simulink model "fs"  (R2020a)
settings: Solver=ode4  StartTime=0.0  StopTime=inf  FixedStep=0.05  RelTol=1e-3
undefined symbols (not defined in the file): Angular, Discrete, Linear, Time
libraries: robotlib x17, simulink x1, ctrlSharedLib x1, dspstat3 x1
settings Model: Creator=ivory  LastModifiedBy=ivory
settings OptimizationCC: EnhancedBackFolding=on  PassReuseOutputArgsAs=Individual arguments  ZeroExternalMemoryAtStartup=off  ZeroInternalMemoryAtStartup=off  MaxStackSize=64  OptimizeBlockOrder=speed  DifferentSizesBufferReuse=on  OptimizationCustomize=off  EfficientTunableParamExpr=on
settings DebuggingCC: ParameterTunabilityLossMsg=error
settings HardwareCC: ProdBitPerPointer=32  ProdBitPerSizeT=32  ProdBitPerPtrDiffT=32  ProdLargestAtomicFloat=None  ProdIntDivRoundTo=Undefined  ProdEndianess=Unspecified  ProdWordSize=32  ProdHWDeviceType=Generic->Unspecified (assume 32-bit Generic)
settings SFSimCC: MATLABDynamicMemAlloc=off
settings RTWCC: SystemTargetFile=ert.tlc  HardwareBoard=Robot Operating System (ROS)  TemplateMakefile=ert_default_tmf  GenerateReport=on  Toolchain=Catkin  IncludeHyperlinkInReport=on  LaunchReport=on  TargetLang=C++  GenerateTraceInfo=on  GenerateTraceReport=on  GenerateTraceReportSl=on  GenerateTraceReportSf=on  GenerateTraceReportEml=on
settings CodeAppCC: ForceParamTrailComments=on  IgnoreCustomStorageClasses=off  OperatorAnnotations=on  SimulinkDataObjDesc=on  SFDataObjDesc=on  InsertBlockDesc=on
settings ERTTargetCC: SupportContinuousTime=on  SupportVariableSizeSignals=on

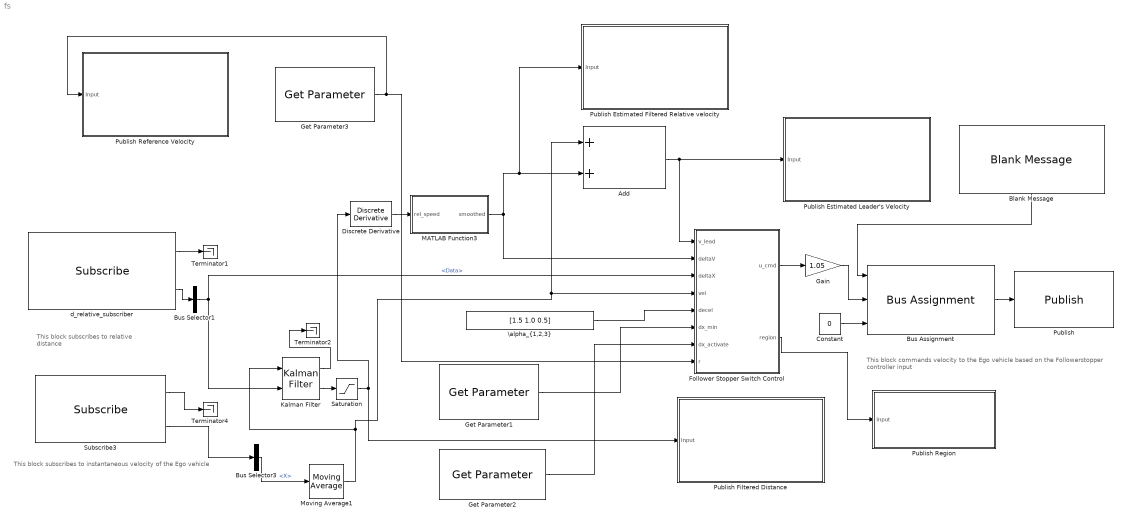
== system fs ==
  note: This block subscribes to
      | instantaneous velocity of the Ego vehicle
  note: This block subscribes
      | to relative distance
  note: This block commands velocity to the Ego vehicle based
      | on the Followerstopper controller input
  Add : Sum
  Blank Message : robotlib/Blank Message  messageClass=Message  entityType=geometry_msgs/Twist  messageType=geometry_msgs/Twist  SampleTime=inf
  Bus Assignment : BusAssignment  AssignedSignals=Linear.X,Angular.Z
  Bus Selector1 : BusSelector  OutputSignals=Data
  Bus Selector3 : BusSelector  OutputSignals=Linear.X
  Constant : Constant  Value=0
  Discrete Derivative : simulink/Discrete/Discrete Derivative  gainval=1  ICPrevScaledInput=15.0  OutMin=[]  OutMax=[]  OutDataType=fixdt(1, 16)  OutScaling=2^-10  RndMeth=Convergent  DoSatur=off
  Follower Stopper Switch Control : Subsystem
  Gain : Gain  Gain=1.05
  Get Parameter1 : robotlib/Get Parameter  ParameterSource=Specify your own  ParameterName=/dx_min  ParameterType=double  ParameterMaxArrayLength=16  ParameterInitialValue=4.5  SampleTime=-1  ShowErrorCodeOutput=off  ModelName=fs  BlockId=ParamGet_fs_35
      settings: SourceProductBaseCode=RR
  Get Parameter2 : robotlib/Get Parameter  ParameterSource=Specify your own  ParameterName=/dx_activate  ParameterType=double  ParameterMaxArrayLength=16  ParameterInitialValue=6.0  SampleTime=-1  ShowErrorCodeOutput=off  ModelName=fs  BlockId=ParamGet_fs_36
      settings: SourceProductBaseCode=RR
  Get Parameter3 : robotlib/Get Parameter  ParameterSource=Specify your own  ParameterName=v_ref  ParameterType=double  ParameterMaxArrayLength=16  ParameterInitialValue=4.5  SampleTime=-1  ShowErrorCodeOutput=off  ModelName=fs  BlockId=ParamGet_fs_161
      settings: SourceProductBaseCode=RR
  Kalman Filter : ctrlSharedLib/Kalman Filter  TimeDomain=Discrete-Time  UseCurrentEstimator=on  ModelSource=LTI State-Space Variable  ModelSourceVariable=ss(-1, 1,1,0, 0.05)  A=0.95  B=1  C=1  D=0  NumberOfStates=1  NumberOfInputs=1  NumberOfOutputs=1  InitialEstimateSource=Dialog  X0=30  P0=10  UseK=off  UseGH=off  NumberOfProcessNoiseInputs=1  G=1  TimeInvariantG=on  H=0  TimeInvariantH=on  Q=0.1  TimeInvariantQ=on  R=0.8  TimeInvariantR=on  N=0  TimeInvariantN=on  AddInputPort=on  AddEnablePort=off  OutputEstimatedY=on  OutputP=off  Ts=-1
  MATLAB Function3 : MATLAB Function  TreatAsAtomicUnit=on
  Moving Average1 : dspstat3/Moving Average  Method=Sliding window  ForgettingFactorPort=off  SpecifyWindowLength=on  WindowLength=20  ForgettingFactor=0.9  SimulateUsing=Code generation
  Publish : robotlib/Publish  topicSource=Specify your own  topic=cmd_vel  messageType=geometry_msgs/Twist  messageQueueLength=1
  Publish Estimated Filtered Relative velocity : Subsystem
  Publish Estimated Leader's Velocity : Subsystem
  Publish Filtered Distance : Subsystem
  Publish Reference Velocity : Subsystem
  Publish Region : Subsystem
  Saturation : Saturate  UpperLimit=252  LowerLimit=0.0
  Subscribe3 : robotlib/Subscribe  topicSource=Specify your own  topic=vel  messageType=geometry_msgs/Twist  sampleTime=-1  messageQueueLength=1
  Terminator1 : Terminator
  Terminator2 : Terminator
  Terminator4 : Terminator
  "\\alpha_{1,2,3}" : Constant  Value=[1.5 1.0 0.5]  OutDataTypeStr=double  SampleTime=-1
  d_relative_subscriber : robotlib/Subscribe  topicSource=Specify your own  topic=d_relative  messageType=std_msgs/Float64  sampleTime=-1  messageQueueLength=1
  wires:
  Bus Assignment/1 -> Publish/1
  d_relative_subscriber/2 -> Bus Selector1/1
  Get Parameter1/1 -> Follower Stopper Switch Control/6(dx_min)
  Subscribe3/2 -> Bus Selector3/1
  Blank Message/1 -> Bus Assignment/1
  Bus Selector3/1 -> Moving Average1/1  "<X>"
  "\\alpha_{1,2,3}"/1 -> Follower Stopper Switch Control/5(decel)
  Get Parameter2/1 -> Follower Stopper Switch Control/7(dx_activate)
  Constant/1 -> Bus Assignment/3
  Subscribe3/1 -> Terminator4/1
  Follower Stopper Switch Control/1(u_cmd) -> Gain/1
  Add/1 -> Follower Stopper Switch Control/1(v_lead), Publish Estimated Leader's Velocity/1(Input)
  Gain/1 -> Bus Assignment/2
  d_relative_subscriber/1 -> Terminator1/1
  Discrete Derivative/1 -> MATLAB Function3/1(rel_speed)
  MATLAB Function3/1(smoothed) -> Publish Estimated Filtered Relative velocity/1(Input), Add/2, Follower Stopper Switch Control/2(deltaV)
  Kalman Filter/2 -> Saturation/1
  Kalman Filter/1 -> Terminator2/1
  Saturation/1 -> Discrete Derivative/1, Publish Filtered Distance/1(Input)
  Bus Selector1/1 -> Kalman Filter/2, Follower Stopper Switch Control/3(deltaX)  "<Data>"
  Moving Average1/1 -> Kalman Filter/1, Follower Stopper Switch Control/4(vel), Add/1
  Follower Stopper Switch Control/2(region) -> Publish Region/1(Input)
  Get Parameter3/1 -> Publish Reference Velocity/1(Input), Follower Stopper Switch Control/8(r)

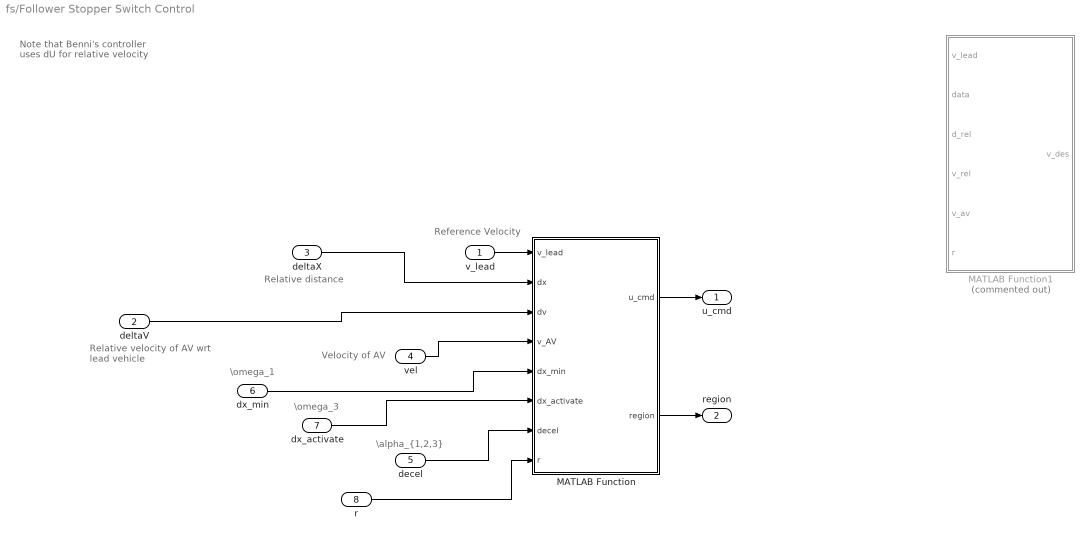
== system fs/Follower Stopper Switch Control ==
  note: Note that Benni's
      | controller uses dU
      | for relative
      | velocity
  note: Relative velocity of
      | AV wrt lead vehicle
  note: Velocity of AV
  note: Reference Velocity
  note: Relative distance
  note: \omega_1
  note: \omega_3
  note: \alpha_{1,2,3}
  v_lead : Inport
  deltaV : Inport  Port=2
  deltaX : Inport  Port=3
  vel : Inport  Port=4
  decel : Inport  Port=5
  dx_min : Inport  Port=6
  dx_activate : Inport  Port=7
  r : Inport  Port=8
  MATLAB Function : MATLAB Function  TreatAsAtomicUnit=on
  MATLAB Function1 : MATLAB Function  Commented=on  TreatAsAtomicUnit=on
  u_cmd : Outport
  region : Outport  Port=2
  wires:
  deltaX/1 -> MATLAB Function/2(dx)
  deltaV/1 -> MATLAB Function/3(dv)
  MATLAB Function/1(u_cmd) -> u_cmd/1
  vel/1 -> MATLAB Function/4(v_AV)
  dx_min/1 -> MATLAB Function/5(dx_min)
  decel/1 -> MATLAB Function/7(decel)
  dx_activate/1 -> MATLAB Function/6(dx_activate)
  v_lead/1 -> MATLAB Function/1(v_lead)
  MATLAB Function/2(region) -> region/1
  r/1 -> MATLAB Function/8(r)

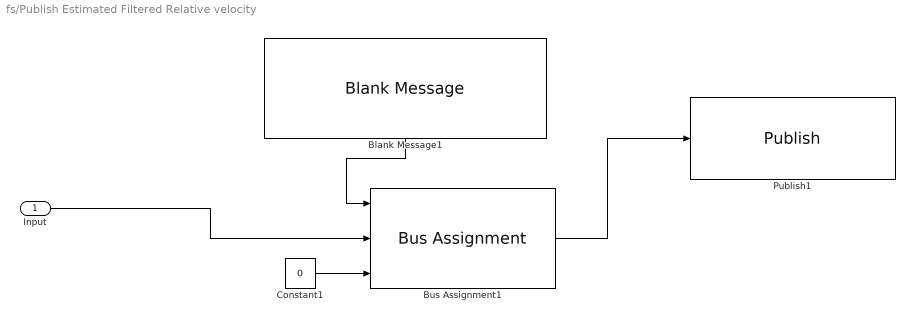
== system fs/Publish Estimated Filtered Relative velocity ==
  Input : Inport
  Blank Message1 : robotlib/Blank Message  messageClass=Message  entityType=geometry_msgs/Twist  messageType=geometry_msgs/Twist  SampleTime=inf
  Bus Assignment1 : BusAssignment  AssignedSignals=Linear.X,Angular.Z
  Constant1 : Constant  Value=0
  Publish1 : robotlib/Publish  topicSource=Specify your own  topic=v_relative_est  messageType=geometry_msgs/Twist  messageQueueLength=1
  wires:
  Input/1 -> Bus Assignment1/2
  Constant1/1 -> Bus Assignment1/3
  Blank Message1/1 -> Bus Assignment1/1
  Bus Assignment1/1 -> Publish1/1

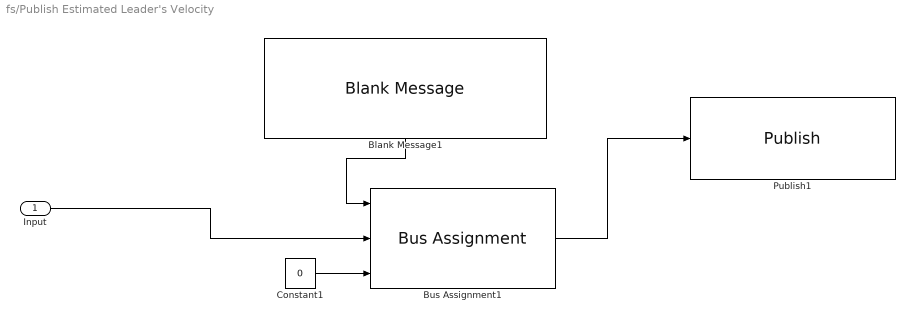
== system fs/Publish Estimated Leader's Velocity ==
  Input : Inport
  Blank Message1 : robotlib/Blank Message  messageClass=Message  entityType=geometry_msgs/Twist  messageType=geometry_msgs/Twist  SampleTime=inf
  Bus Assignment1 : BusAssignment  AssignedSignals=Linear.X,Angular.Z
  Constant1 : Constant  Value=0
  Publish1 : robotlib/Publish  topicSource=Specify your own  topic=v_leader_est  messageType=geometry_msgs/Twist  messageQueueLength=1
  wires:
  Bus Assignment1/1 -> Publish1/1
  Blank Message1/1 -> Bus Assignment1/1
  Constant1/1 -> Bus Assignment1/3
  Input/1 -> Bus Assignment1/2

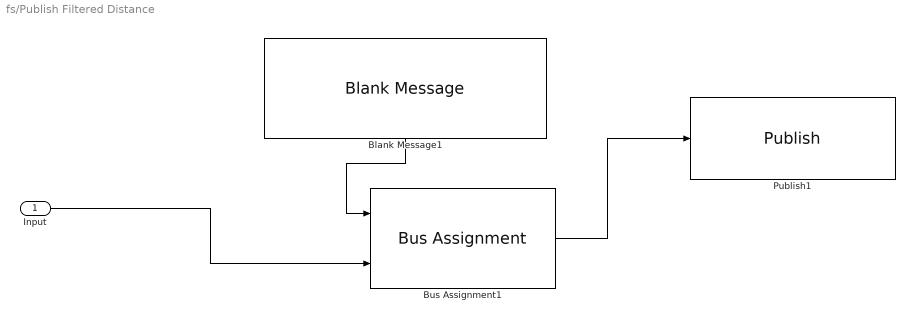
== system fs/Publish Filtered Distance ==
  Input : Inport
  Blank Message1 : robotlib/Blank Message  messageClass=Message  entityType=std_msgs/Float64  messageType=std_msgs/Float64  SampleTime=inf
  Bus Assignment1 : BusAssignment  AssignedSignals=Data
  Publish1 : robotlib/Publish  topicSource=Specify your own  topic=distance_filtered  messageType=std_msgs/Float64  messageQueueLength=1
  wires:
  Input/1 -> Bus Assignment1/2
  Blank Message1/1 -> Bus Assignment1/1
  Bus Assignment1/1 -> Publish1/1

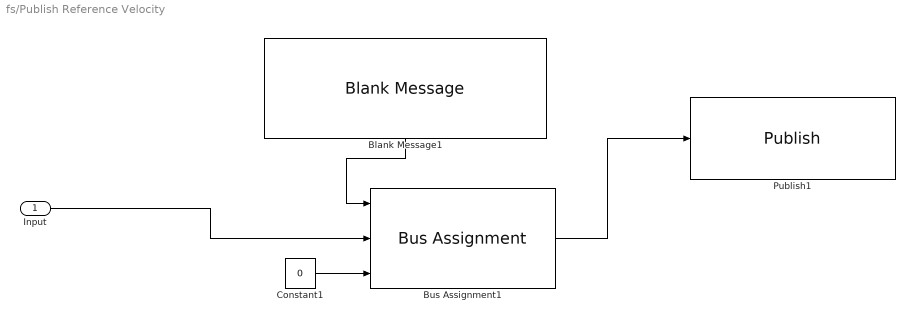
== system fs/Publish Reference Velocity ==
  Input : Inport
  Blank Message1 : robotlib/Blank Message  messageClass=Message  entityType=geometry_msgs/Twist  messageType=geometry_msgs/Twist  SampleTime=inf
  Bus Assignment1 : BusAssignment  AssignedSignals=Linear.X,Angular.Z
  Constant1 : Constant  Value=0
  Publish1 : robotlib/Publish  topicSource=Specify your own  topic=velocity_ref  messageType=geometry_msgs/Twist  messageQueueLength=1
  wires:
  Input/1 -> Bus Assignment1/2
  Constant1/1 -> Bus Assignment1/3
  Blank Message1/1 -> Bus Assignment1/1
  Bus Assignment1/1 -> Publish1/1

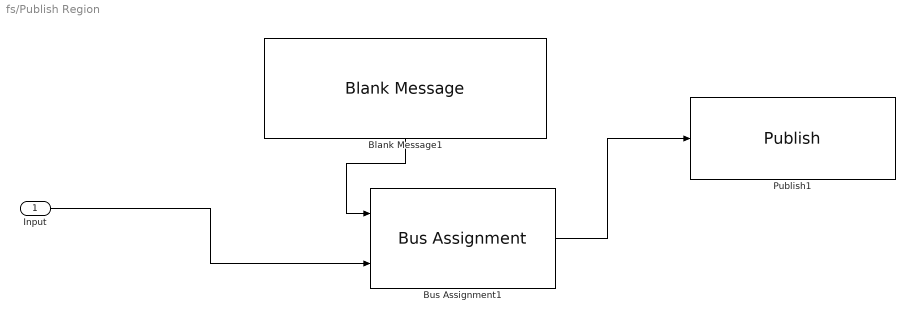
== system fs/Publish Region ==
  Input : Inport
  Blank Message1 : robotlib/Blank Message  messageClass=Message  entityType=std_msgs/UInt8  messageType=std_msgs/UInt8  SampleTime=inf
  Bus Assignment1 : BusAssignment  AssignedSignals=Data
  Publish1 : robotlib/Publish  topicSource=Specify your own  topic=region  messageType=std_msgs/UInt8  messageQueueLength=1
  wires:
  Input/1 -> Bus Assignment1/2
  Blank Message1/1 -> Bus Assignment1/1
  Bus Assignment1/1 -> Publish1/1

== matlab function fs/Follower Stopper Switch Control/MATLAB Function1 ==
  data: v_lead input; data input; v_des output; d_rel input; v_rel input; v_av input; r input
function v_des = fcn(v_lead, data, d_rel,v_rel,v_av, r)
%#codegen
% Safety controller, based on quadratic bands.
% Input: r = desired velocity (from other models)
%          d_rel = estimate of gap to vehicle ahead
%          v_rel = estimate of time derivative of dx (= velocity difference)
%         v_AV = velocity of AV
%      dx_min = minimum distance
% dx_activate = distance below which controller does something
%       decel = vector of three deceleration values for parabolas
% Out:  u_cmd = actual velocity commanded (always u_cmd<=U)
%
% Controller-specific parameters

    w = zeros(3,1);
    alpha = zeros(3,1);
    w(1) = 4.5;
    alpha(1) = 1.5;
    w(3) = 6.0;
    alpha(3) = 0.5;
    w(2) = (w(1)+w(3))/2;
    alpha(2) = (alpha(1)+alpha(3))/2;
    if(nargin<4)
        r = 30;
    end
    
    %v_rel_star = min(v_rel,0)
    v_rel_star = v_rel;
    v_rel_star(v_rel >= 0) = 0;
   
    h_1 = 0.4;
    h_2 = 1.2;
    h_3 = 1.8;
    
    x1 = w(1) + (0.5*v_rel_star.^2)/alpha(1) + h_1*v_av;
    x2 = w(2) + (0.5*v_rel_star.^2)/alpha(2) + h_2*v_av;
    x3 = w(3) + (0.5*v_rel_star.^2)/alpha(3) + h_3*v_av;
    
%     v_lead = v_av+v_rel;
    
    
    %v = min([max([v_lead,0]),r]);
    v = v_lead;
    v(v_lead<0) = 0;
    
    v(v_lead>r) = r;
  
    v_des = zeros(size(d_rel));  
    %safe region
    v_des(d_rel>x3) = r;  
    %adaptation region 1
    temp_v_des = v+(r-v).*(d_rel-x2)./(x3-x2);
    v_des(d_rel>x2 & d_rel<=x3) = temp_v_des(d_rel>x2 & d_rel<=x3);   
    %adaptation region 2
    temp_v_des = v.*(d_rel-x1)./(x2-x1);
    v_des(d_rel>x1 & d_rel<=x2) = temp_v_des(d_rel>x1 & d_rel<=x2);

== matlab function fs/MATLAB Function3 ==
  data: rel_speed input; smoothed output
function  smoothed = online_smoothing(rel_speed)

array_length = 75;
window_size = 70;
persistent array

persistent count

if isempty(count)
    count = 0;
else
    
    if count < 75
        count = count + 1;
    end
    
end

if isempty(array)
    array = zeros(1, array_length);
else
    array = [array(2:end), rel_speed];
end

if count < 70
    smoothed = rel_speed;
else
    smoothed_array = smoothdata(array, 'sgolay',window_size);
    smoothed = smoothed_array(end);
end

== matlab function fs/Follower Stopper Switch Control/MATLAB Function ==
  data: v_lead input; u_cmd output; dx input; dv input; v_AV input; dx_min input; dx_activate input; decel input; region output; r input
function [u_cmd, region] = fcn(v_lead, dx,dv,v_AV,...
    dx_min,dx_activate,decel, r)
%#codegen
% Safety controller, based on quadratic bands.
% Input: r = desired velocity (from other models)
%          dx = estimate of gap to vehicle ahead
%          dv = estimate of time derivative of dx (= velocity difference)
%         v_AV = velocity of AV
%      dx_min = minimum distance
% dx_activate = distance below which controller does something
%       decel = vector of three deceleration values for parabolas
% Out:  u_cmd = actual velocity commanded (always u_cmd<=U)
%
% Controller-specific parameters
dx_mid = (dx_min+dx_activate)/2; % mid distance, where v_lead is commanded
% Lead vehicle velocity
%v_lead = v_AV+dv; % velocity of lead vehicle
%r = v_lead;
v_lead = max(v_lead,0); % lead vehicle cannot go backwards
v = min(r,v_lead); % safety velocity cannot exceed desired velocity U
% Treatment of positive dv-values
dv = min(dv,0); % domains for dv>0 same as dv=0
% For given dv, dx-values of band boundaries
dx1 = dx_min+1/(2*decel(1))*dv.^2;
dx2 = dx_mid+1/(2*decel(2))*dv.^2;
dx3 = dx_activate+1/(2*decel(3))*dv.^2;
% Actual commanded velocity
u_cmd = double((dx1<dx&dx<=dx2).*(v.*(dx-dx1)./(dx2-dx1))+...
    (dx2<dx&dx<=dx3).*(v+(r-v).*(dx-dx2)./(dx3-dx2))+...
    (dx3<dx).*r);
% DO not move if within dx_min
% if(dx < dx_min)
%     u_cmd = 0;
% end

if( dx > 16.0 )
    u_cmd = r;
end

if dx>dx3
        region = uint8(0);
    elseif dx>dx2 && dx<=dx3
        region = uint8(1);
    elseif dx>dx1 && dx<=dx2
        region = uint8(2);
    else
        region = uint8(3);
    end
